simulink library "Computer_Library"  (Simulink 8.1)
settings: Solver=ode45  StartTime=0.0  StopTime=10.0  RelTol=1e-3
values from neighbouring files (symbols this model uses):
  A = 10    [CharTable.m]
  ARROW_DOWN = 48    [CharTable.m]
  ARROW_LEFT = 49    [CharTable.m]
  ARROW_RIGHT = 50    [CharTable.m]
  ARROW_UP = 47    [CharTable.m]
  ASTERISK = 39    [CharTable.m]
  B = 11    [CharTable.m]
  BACKSLASH = 43    [CharTable.m]
  C = 12    [CharTable.m]
  COLON = 40    [CharTable.m]
  COMMA = 53    [CharTable.m]
  CROSS = 38    [CharTable.m]
  CURSOR = 62    [CharTable.m]
  D = 13    [CharTable.m]
  DOT = 52    [CharTable.m]
  EQUAL = 44    [CharTable.m]
  EXCLAMATION_MARK = 55    [CharTable.m]
  F = 15    [CharTable.m]
  G = 16    [CharTable.m]
  GREATER_THAN = 46    [CharTable.m]
  H = 17    [CharTable.m]
  I = 18    [CharTable.m]
  J = 19    [CharTable.m]
  K = 20    [CharTable.m]
  L = 21    [CharTable.m]
  LEFT_PARENTHESES = 59    [CharTable.m]
  LESS_THAN = 45    [CharTable.m]
  M = 22    [CharTable.m]
  MINUS = 37    [CharTable.m]
  N = 23    [CharTable.m]
  O = 24    [CharTable.m]
  P = 25    [CharTable.m]
  PERCENT = 58    [CharTable.m]
  PLUS = 36    [CharTable.m]
  Q = 32    [CharTable.m]
  QUESTION_MARK = 54    [CharTable.m]
  QUOTE = 56    [CharTable.m]
  R = 26    [CharTable.m]
  RECTANGLE = 63    [CharTable.m]
  RIGHT_PARENTHESES = 60    [CharTable.m]
  RomCode = reshape(transpose(RomCode), [], 1)    [ROM.m]
  S = 27    [CharTable.m]
  SEMICOLON = 41    [CharTable.m]
  SHARP = 57    [CharTable.m]
  SLASH = 42    [CharTable.m]
  SPACE = 61    [CharTable.m]
  T = 28    [CharTable.m]
  U = 29    [CharTable.m]
  UNDERSCORE = 51    [CharTable.m]
  V = 30    [CharTable.m]
  W = 31    [CharTable.m]
  X = 33    [CharTable.m]
  Y = 34    [CharTable.m]
  Z = 35    [CharTable.m]
undefined symbols (not defined in the file or in its folder): char_0
libraries: Memory_Blocks_Lib x116, Byte_Multiplexers_Lib x44, commutil2 x18, Bit_Multiplexers_Lib x17, Decoders_Lib x9, simulink_extras x8, Logic_Operations_Lib x4, Byte_Demultiplexers_Lib x2, Arithmetic_Operations_Lib x2, dspsnks4 x1
(part 4 of 4)

== system Computer_Library/Character_Table/Characters(ARROW_DOWN..RECTANGLE)/Char_QUOTE ==
  Byte_01 : Constant  Value=char(2, QUOTE)  OutDataTypeStr=uint8
  Byte_02 : Constant  Value=char(3, QUOTE)  OutDataTypeStr=uint8
  Byte_03 : Constant  Value=char(4, QUOTE)  OutDataTypeStr=uint8
  Byte_04 : Constant  Value=char(5, QUOTE)  OutDataTypeStr=uint8
  Byte_05 : Constant  Value=char(6, QUOTE)  OutDataTypeStr=uint8
  Byte_06 : Constant  Value=char(7, QUOTE)  OutDataTypeStr=uint8
  Byte_07 : Constant  Value=char(8, QUOTE)  OutDataTypeStr=uint8
  Byte_1 : Constant  Value=char(1, QUOTE)  OutDataTypeStr=uint8
  Column_1(1B) : Outport
  Column_2(1B) : Outport  Port=2
  Column_3(1B) : Outport  Port=3
  Column_4(1B) : Outport  Port=4
  Column_5(1B) : Outport  Port=5
  Column_6(1B) : Outport  Port=6
  Column_7(1B) : Outport  Port=7
  Column_8(1B) : Outport  Port=8
  wires:
  Byte_05/1 -> Column_6(1B)/1
  Byte_04/1 -> Column_5(1B)/1
  Byte_01/1 -> Column_2(1B)/1
  Byte_07/1 -> Column_8(1B)/1
  Byte_03/1 -> Column_4(1B)/1
  Byte_06/1 -> Column_7(1B)/1
  Byte_1/1 -> Column_1(1B)/1
  Byte_02/1 -> Column_3(1B)/1

== system Computer_Library/Character_Table/Characters(ARROW_DOWN..RECTANGLE)/Char_RECTANGLE ==
  Byte_01 : Constant  Value=char(2, RECTANGLE)  OutDataTypeStr=uint8
  Byte_02 : Constant  Value=char(3, RECTANGLE)  OutDataTypeStr=uint8
  Byte_03 : Constant  Value=char(4, RECTANGLE)  OutDataTypeStr=uint8
  Byte_04 : Constant  Value=char(5, RECTANGLE)  OutDataTypeStr=uint8
  Byte_05 : Constant  Value=char(6, RECTANGLE)  OutDataTypeStr=uint8
  Byte_06 : Constant  Value=char(7, RECTANGLE)  OutDataTypeStr=uint8
  Byte_07 : Constant  Value=char(8, RECTANGLE)  OutDataTypeStr=uint8
  Byte_1 : Constant  Value=char(1, RECTANGLE)  OutDataTypeStr=uint8
  Column_1(1B) : Outport
  Column_2(1B) : Outport  Port=2
  Column_3(1B) : Outport  Port=3
  Column_4(1B) : Outport  Port=4
  Column_5(1B) : Outport  Port=5
  Column_6(1B) : Outport  Port=6
  Column_7(1B) : Outport  Port=7
  Column_8(1B) : Outport  Port=8
  wires:
  Byte_05/1 -> Column_6(1B)/1
  Byte_04/1 -> Column_5(1B)/1
  Byte_01/1 -> Column_2(1B)/1
  Byte_07/1 -> Column_8(1B)/1
  Byte_03/1 -> Column_4(1B)/1
  Byte_06/1 -> Column_7(1B)/1
  Byte_1/1 -> Column_1(1B)/1
  Byte_02/1 -> Column_3(1B)/1

== system Computer_Library/Character_Table/Characters(ARROW_DOWN..RECTANGLE)/Char_RIGHT_PARENTHESES ==
  Byte_01 : Constant  Value=char(2, RIGHT_PARENTHESES)  OutDataTypeStr=uint8
  Byte_02 : Constant  Value=char(3, RIGHT_PARENTHESES)  OutDataTypeStr=uint8
  Byte_03 : Constant  Value=char(4, RIGHT_PARENTHESES)  OutDataTypeStr=uint8
  Byte_04 : Constant  Value=char(5, RIGHT_PARENTHESES)  OutDataTypeStr=uint8
  Byte_05 : Constant  Value=char(6, RIGHT_PARENTHESES)  OutDataTypeStr=uint8
  Byte_06 : Constant  Value=char(7, RIGHT_PARENTHESES)  OutDataTypeStr=uint8
  Byte_07 : Constant  Value=char(8, RIGHT_PARENTHESES)  OutDataTypeStr=uint8
  Byte_1 : Constant  Value=char(1, RIGHT_PARENTHESES)  OutDataTypeStr=uint8
  Column_1(1B) : Outport
  Column_2(1B) : Outport  Port=2
  Column_3(1B) : Outport  Port=3
  Column_4(1B) : Outport  Port=4
  Column_5(1B) : Outport  Port=5
  Column_6(1B) : Outport  Port=6
  Column_7(1B) : Outport  Port=7
  Column_8(1B) : Outport  Port=8
  wires:
  Byte_05/1 -> Column_6(1B)/1
  Byte_04/1 -> Column_5(1B)/1
  Byte_01/1 -> Column_2(1B)/1
  Byte_07/1 -> Column_8(1B)/1
  Byte_03/1 -> Column_4(1B)/1
  Byte_06/1 -> Column_7(1B)/1
  Byte_1/1 -> Column_1(1B)/1
  Byte_02/1 -> Column_3(1B)/1

== system Computer_Library/Character_Table/Characters(ARROW_DOWN..RECTANGLE)/Char_SHARP ==
  Byte_01 : Constant  Value=char(2, SHARP)  OutDataTypeStr=uint8
  Byte_02 : Constant  Value=char(3, SHARP)  OutDataTypeStr=uint8
  Byte_03 : Constant  Value=char(4, SHARP)  OutDataTypeStr=uint8
  Byte_04 : Constant  Value=char(5, SHARP)  OutDataTypeStr=uint8
  Byte_05 : Constant  Value=char(6, SHARP)  OutDataTypeStr=uint8
  Byte_06 : Constant  Value=char(7, SHARP)  OutDataTypeStr=uint8
  Byte_07 : Constant  Value=char(8, SHARP)  OutDataTypeStr=uint8
  Byte_1 : Constant  Value=char(1, SHARP)  OutDataTypeStr=uint8
  Column_1(1B) : Outport
  Column_2(1B) : Outport  Port=2
  Column_3(1B) : Outport  Port=3
  Column_4(1B) : Outport  Port=4
  Column_5(1B) : Outport  Port=5
  Column_6(1B) : Outport  Port=6
  Column_7(1B) : Outport  Port=7
  Column_8(1B) : Outport  Port=8
  wires:
  Byte_05/1 -> Column_6(1B)/1
  Byte_04/1 -> Column_5(1B)/1
  Byte_01/1 -> Column_2(1B)/1
  Byte_07/1 -> Column_8(1B)/1
  Byte_03/1 -> Column_4(1B)/1
  Byte_06/1 -> Column_7(1B)/1
  Byte_1/1 -> Column_1(1B)/1
  Byte_02/1 -> Column_3(1B)/1

== system Computer_Library/Character_Table/Characters(ARROW_DOWN..RECTANGLE)/Char_SPACE ==
  Byte_01 : Constant  Value=char(2, SPACE)  OutDataTypeStr=uint8
  Byte_02 : Constant  Value=char(3, SPACE)  OutDataTypeStr=uint8
  Byte_03 : Constant  Value=char(4, SPACE)  OutDataTypeStr=uint8
  Byte_04 : Constant  Value=char(5, SPACE)  OutDataTypeStr=uint8
  Byte_05 : Constant  Value=char(6, SPACE)  OutDataTypeStr=uint8
  Byte_06 : Constant  Value=char(7, SPACE)  OutDataTypeStr=uint8
  Byte_07 : Constant  Value=char(8, SPACE)  OutDataTypeStr=uint8
  Byte_1 : Constant  Value=char(1, SPACE)  OutDataTypeStr=uint8
  Column_1(1B) : Outport
  Column_2(1B) : Outport  Port=2
  Column_3(1B) : Outport  Port=3
  Column_4(1B) : Outport  Port=4
  Column_5(1B) : Outport  Port=5
  Column_6(1B) : Outport  Port=6
  Column_7(1B) : Outport  Port=7
  Column_8(1B) : Outport  Port=8
  wires:
  Byte_05/1 -> Column_6(1B)/1
  Byte_04/1 -> Column_5(1B)/1
  Byte_01/1 -> Column_2(1B)/1
  Byte_07/1 -> Column_8(1B)/1
  Byte_03/1 -> Column_4(1B)/1
  Byte_06/1 -> Column_7(1B)/1
  Byte_1/1 -> Column_1(1B)/1
  Byte_02/1 -> Column_3(1B)/1

== system Computer_Library/Character_Table/Characters(ARROW_DOWN..RECTANGLE)/Char_UNDERSCORE ==
  Byte_01 : Constant  Value=char(2, UNDERSCORE)  OutDataTypeStr=uint8
  Byte_02 : Constant  Value=char(3, UNDERSCORE)  OutDataTypeStr=uint8
  Byte_03 : Constant  Value=char(4, UNDERSCORE)  OutDataTypeStr=uint8
  Byte_04 : Constant  Value=char(5, UNDERSCORE)  OutDataTypeStr=uint8
  Byte_05 : Constant  Value=char(6, UNDERSCORE)  OutDataTypeStr=uint8
  Byte_06 : Constant  Value=char(7, UNDERSCORE)  OutDataTypeStr=uint8
  Byte_07 : Constant  Value=char(8, UNDERSCORE)  OutDataTypeStr=uint8
  Byte_1 : Constant  Value=char(1, UNDERSCORE)  OutDataTypeStr=uint8
  Column_1(1B) : Outport
  Column_2(1B) : Outport  Port=2
  Column_3(1B) : Outport  Port=3
  Column_4(1B) : Outport  Port=4
  Column_5(1B) : Outport  Port=5
  Column_6(1B) : Outport  Port=6
  Column_7(1B) : Outport  Port=7
  Column_8(1B) : Outport  Port=8
  wires:
  Byte_05/1 -> Column_6(1B)/1
  Byte_04/1 -> Column_5(1B)/1
  Byte_01/1 -> Column_2(1B)/1
  Byte_07/1 -> Column_8(1B)/1
  Byte_03/1 -> Column_4(1B)/1
  Byte_06/1 -> Column_7(1B)/1
  Byte_1/1 -> Column_1(1B)/1
  Byte_02/1 -> Column_3(1B)/1

== system Computer_Library/Character_Table/Characters(G..W)/Char_G ==
  Byte_01 : Constant  Value=char(2, G)  OutDataTypeStr=uint8
  Byte_02 : Constant  Value=char(3, G)  OutDataTypeStr=uint8
  Byte_03 : Constant  Value=char(4, G)  OutDataTypeStr=uint8
  Byte_04 : Constant  Value=char(5, G)  OutDataTypeStr=uint8
  Byte_05 : Constant  Value=char(6, G)  OutDataTypeStr=uint8
  Byte_06 : Constant  Value=char(7, G)  OutDataTypeStr=uint8
  Byte_07 : Constant  Value=char(8, G)  OutDataTypeStr=uint8
  Byte_1 : Constant  Value=char(1, G)  OutDataTypeStr=uint8
  Column_1(1B) : Outport
  Column_2(1B) : Outport  Port=2
  Column_3(1B) : Outport  Port=3
  Column_4(1B) : Outport  Port=4
  Column_5(1B) : Outport  Port=5
  Column_6(1B) : Outport  Port=6
  Column_7(1B) : Outport  Port=7
  Column_8(1B) : Outport  Port=8
  wires:
  Byte_05/1 -> Column_6(1B)/1
  Byte_04/1 -> Column_5(1B)/1
  Byte_01/1 -> Column_2(1B)/1
  Byte_07/1 -> Column_8(1B)/1
  Byte_03/1 -> Column_4(1B)/1
  Byte_06/1 -> Column_7(1B)/1
  Byte_1/1 -> Column_1(1B)/1
  Byte_02/1 -> Column_3(1B)/1

== system Computer_Library/Character_Table/Characters(G..W)/Char_H ==
  Byte_01 : Constant  Value=char(2, H)  OutDataTypeStr=uint8
  Byte_02 : Constant  Value=char(3, H)  OutDataTypeStr=uint8
  Byte_03 : Constant  Value=char(4, H)  OutDataTypeStr=uint8
  Byte_04 : Constant  Value=char(5, H)  OutDataTypeStr=uint8
  Byte_05 : Constant  Value=char(6, H)  OutDataTypeStr=uint8
  Byte_06 : Constant  Value=char(7, H)  OutDataTypeStr=uint8
  Byte_07 : Constant  Value=char(8, H)  OutDataTypeStr=uint8
  Byte_1 : Constant  Value=char(1, H)  OutDataTypeStr=uint8
  Column_1(1B) : Outport
  Column_2(1B) : Outport  Port=2
  Column_3(1B) : Outport  Port=3
  Column_4(1B) : Outport  Port=4
  Column_5(1B) : Outport  Port=5
  Column_6(1B) : Outport  Port=6
  Column_7(1B) : Outport  Port=7
  Column_8(1B) : Outport  Port=8
  wires:
  Byte_05/1 -> Column_6(1B)/1
  Byte_04/1 -> Column_5(1B)/1
  Byte_01/1 -> Column_2(1B)/1
  Byte_07/1 -> Column_8(1B)/1
  Byte_03/1 -> Column_4(1B)/1
  Byte_06/1 -> Column_7(1B)/1
  Byte_1/1 -> Column_1(1B)/1
  Byte_02/1 -> Column_3(1B)/1

== system Computer_Library/Character_Table/Characters(G..W)/Char_I ==
  Byte_01 : Constant  Value=char(2, I)  OutDataTypeStr=uint8
  Byte_02 : Constant  Value=char(3, I)  OutDataTypeStr=uint8
  Byte_03 : Constant  Value=char(4, I)  OutDataTypeStr=uint8
  Byte_04 : Constant  Value=char(5, I)  OutDataTypeStr=uint8
  Byte_05 : Constant  Value=char(6, I)  OutDataTypeStr=uint8
  Byte_06 : Constant  Value=char(7, I)  OutDataTypeStr=uint8
  Byte_07 : Constant  Value=char(8, I)  OutDataTypeStr=uint8
  Byte_1 : Constant  Value=char(1, I)  OutDataTypeStr=uint8
  Column_1(1B) : Outport
  Column_2(1B) : Outport  Port=2
  Column_3(1B) : Outport  Port=3
  Column_4(1B) : Outport  Port=4
  Column_5(1B) : Outport  Port=5
  Column_6(1B) : Outport  Port=6
  Column_7(1B) : Outport  Port=7
  Column_8(1B) : Outport  Port=8
  wires:
  Byte_05/1 -> Column_6(1B)/1
  Byte_04/1 -> Column_5(1B)/1
  Byte_01/1 -> Column_2(1B)/1
  Byte_07/1 -> Column_8(1B)/1
  Byte_03/1 -> Column_4(1B)/1
  Byte_06/1 -> Column_7(1B)/1
  Byte_1/1 -> Column_1(1B)/1
  Byte_02/1 -> Column_3(1B)/1

== system Computer_Library/Character_Table/Characters(G..W)/Char_J ==
  Byte_01 : Constant  Value=char(2, J)  OutDataTypeStr=uint8
  Byte_02 : Constant  Value=char(3, J)  OutDataTypeStr=uint8
  Byte_03 : Constant  Value=char(4, J)  OutDataTypeStr=uint8
  Byte_04 : Constant  Value=char(5, J)  OutDataTypeStr=uint8
  Byte_05 : Constant  Value=char(6, J)  OutDataTypeStr=uint8
  Byte_06 : Constant  Value=char(7, J)  OutDataTypeStr=uint8
  Byte_07 : Constant  Value=char(8, J)  OutDataTypeStr=uint8
  Byte_1 : Constant  Value=char(1, J)  OutDataTypeStr=uint8
  Column_1(1B) : Outport
  Column_2(1B) : Outport  Port=2
  Column_3(1B) : Outport  Port=3
  Column_4(1B) : Outport  Port=4
  Column_5(1B) : Outport  Port=5
  Column_6(1B) : Outport  Port=6
  Column_7(1B) : Outport  Port=7
  Column_8(1B) : Outport  Port=8
  wires:
  Byte_05/1 -> Column_6(1B)/1
  Byte_04/1 -> Column_5(1B)/1
  Byte_01/1 -> Column_2(1B)/1
  Byte_07/1 -> Column_8(1B)/1
  Byte_03/1 -> Column_4(1B)/1
  Byte_06/1 -> Column_7(1B)/1
  Byte_1/1 -> Column_1(1B)/1
  Byte_02/1 -> Column_3(1B)/1

== system Computer_Library/Character_Table/Characters(G..W)/Char_K ==
  Byte_01 : Constant  Value=char(2, K)  OutDataTypeStr=uint8
  Byte_02 : Constant  Value=char(3, K)  OutDataTypeStr=uint8
  Byte_03 : Constant  Value=char(4, K)  OutDataTypeStr=uint8
  Byte_04 : Constant  Value=char(5, K)  OutDataTypeStr=uint8
  Byte_05 : Constant  Value=char(6, K)  OutDataTypeStr=uint8
  Byte_06 : Constant  Value=char(7, K)  OutDataTypeStr=uint8
  Byte_07 : Constant  Value=char(8, K)  OutDataTypeStr=uint8
  Byte_1 : Constant  Value=char(1, K)  OutDataTypeStr=uint8
  Column_1(1B) : Outport
  Column_2(1B) : Outport  Port=2
  Column_3(1B) : Outport  Port=3
  Column_4(1B) : Outport  Port=4
  Column_5(1B) : Outport  Port=5
  Column_6(1B) : Outport  Port=6
  Column_7(1B) : Outport  Port=7
  Column_8(1B) : Outport  Port=8
  wires:
  Byte_05/1 -> Column_6(1B)/1
  Byte_04/1 -> Column_5(1B)/1
  Byte_01/1 -> Column_2(1B)/1
  Byte_07/1 -> Column_8(1B)/1
  Byte_03/1 -> Column_4(1B)/1
  Byte_06/1 -> Column_7(1B)/1
  Byte_1/1 -> Column_1(1B)/1
  Byte_02/1 -> Column_3(1B)/1

== system Computer_Library/Character_Table/Characters(G..W)/Char_L ==
  Byte_01 : Constant  Value=char(2, L)  OutDataTypeStr=uint8
  Byte_02 : Constant  Value=char(3, L)  OutDataTypeStr=uint8
  Byte_03 : Constant  Value=char(4, L)  OutDataTypeStr=uint8
  Byte_04 : Constant  Value=char(5, L)  OutDataTypeStr=uint8
  Byte_05 : Constant  Value=char(6, L)  OutDataTypeStr=uint8
  Byte_06 : Constant  Value=char(7, L)  OutDataTypeStr=uint8
  Byte_07 : Constant  Value=char(8, L)  OutDataTypeStr=uint8
  Byte_1 : Constant  Value=char(1, L)  OutDataTypeStr=uint8
  Column_1(1B) : Outport
  Column_2(1B) : Outport  Port=2
  Column_3(1B) : Outport  Port=3
  Column_4(1B) : Outport  Port=4
  Column_5(1B) : Outport  Port=5
  Column_6(1B) : Outport  Port=6
  Column_7(1B) : Outport  Port=7
  Column_8(1B) : Outport  Port=8
  wires:
  Byte_05/1 -> Column_6(1B)/1
  Byte_04/1 -> Column_5(1B)/1
  Byte_01/1 -> Column_2(1B)/1
  Byte_07/1 -> Column_8(1B)/1
  Byte_03/1 -> Column_4(1B)/1
  Byte_06/1 -> Column_7(1B)/1
  Byte_1/1 -> Column_1(1B)/1
  Byte_02/1 -> Column_3(1B)/1

== system Computer_Library/Character_Table/Characters(G..W)/Char_M ==
  Byte_01 : Constant  Value=char(2, M)  OutDataTypeStr=uint8
  Byte_02 : Constant  Value=char(3, M)  OutDataTypeStr=uint8
  Byte_03 : Constant  Value=char(4, M)  OutDataTypeStr=uint8
  Byte_04 : Constant  Value=char(5, M)  OutDataTypeStr=uint8
  Byte_05 : Constant  Value=char(6, M)  OutDataTypeStr=uint8
  Byte_06 : Constant  Value=char(7, M)  OutDataTypeStr=uint8
  Byte_07 : Constant  Value=char(8, M)  OutDataTypeStr=uint8
  Byte_1 : Constant  Value=char(1, M)  OutDataTypeStr=uint8
  Column_1(1B) : Outport
  Column_2(1B) : Outport  Port=2
  Column_3(1B) : Outport  Port=3
  Column_4(1B) : Outport  Port=4
  Column_5(1B) : Outport  Port=5
  Column_6(1B) : Outport  Port=6
  Column_7(1B) : Outport  Port=7
  Column_8(1B) : Outport  Port=8
  wires:
  Byte_05/1 -> Column_6(1B)/1
  Byte_04/1 -> Column_5(1B)/1
  Byte_01/1 -> Column_2(1B)/1
  Byte_07/1 -> Column_8(1B)/1
  Byte_03/1 -> Column_4(1B)/1
  Byte_06/1 -> Column_7(1B)/1
  Byte_1/1 -> Column_1(1B)/1
  Byte_02/1 -> Column_3(1B)/1

== system Computer_Library/Character_Table/Characters(G..W)/Char_N ==
  Byte_01 : Constant  Value=char(2, N)  OutDataTypeStr=uint8
  Byte_02 : Constant  Value=char(3, N)  OutDataTypeStr=uint8
  Byte_03 : Constant  Value=char(4, N)  OutDataTypeStr=uint8
  Byte_04 : Constant  Value=char(5, N)  OutDataTypeStr=uint8
  Byte_05 : Constant  Value=char(6, N)  OutDataTypeStr=uint8
  Byte_06 : Constant  Value=char(7, N)  OutDataTypeStr=uint8
  Byte_07 : Constant  Value=char(8, N)  OutDataTypeStr=uint8
  Byte_1 : Constant  Value=char(1, N)  OutDataTypeStr=uint8
  Column_1(1B) : Outport
  Column_2(1B) : Outport  Port=2
  Column_3(1B) : Outport  Port=3
  Column_4(1B) : Outport  Port=4
  Column_5(1B) : Outport  Port=5
  Column_6(1B) : Outport  Port=6
  Column_7(1B) : Outport  Port=7
  Column_8(1B) : Outport  Port=8
  wires:
  Byte_05/1 -> Column_6(1B)/1
  Byte_04/1 -> Column_5(1B)/1
  Byte_01/1 -> Column_2(1B)/1
  Byte_07/1 -> Column_8(1B)/1
  Byte_03/1 -> Column_4(1B)/1
  Byte_06/1 -> Column_7(1B)/1
  Byte_1/1 -> Column_1(1B)/1
  Byte_02/1 -> Column_3(1B)/1

== system Computer_Library/Character_Table/Characters(G..W)/Char_O ==
  Byte_01 : Constant  Value=char(2, O)  OutDataTypeStr=uint8
  Byte_02 : Constant  Value=char(3, O)  OutDataTypeStr=uint8
  Byte_03 : Constant  Value=char(4, O)  OutDataTypeStr=uint8
  Byte_04 : Constant  Value=char(5, O)  OutDataTypeStr=uint8
  Byte_05 : Constant  Value=char(6, O)  OutDataTypeStr=uint8
  Byte_06 : Constant  Value=char(7, O)  OutDataTypeStr=uint8
  Byte_07 : Constant  Value=char(8, O)  OutDataTypeStr=uint8
  Byte_1 : Constant  Value=char(1, O)  OutDataTypeStr=uint8
  Column_1(1B) : Outport
  Column_2(1B) : Outport  Port=2
  Column_3(1B) : Outport  Port=3
  Column_4(1B) : Outport  Port=4
  Column_5(1B) : Outport  Port=5
  Column_6(1B) : Outport  Port=6
  Column_7(1B) : Outport  Port=7
  Column_8(1B) : Outport  Port=8
  wires:
  Byte_05/1 -> Column_6(1B)/1
  Byte_04/1 -> Column_5(1B)/1
  Byte_01/1 -> Column_2(1B)/1
  Byte_07/1 -> Column_8(1B)/1
  Byte_03/1 -> Column_4(1B)/1
  Byte_06/1 -> Column_7(1B)/1
  Byte_1/1 -> Column_1(1B)/1
  Byte_02/1 -> Column_3(1B)/1

== system Computer_Library/Character_Table/Characters(G..W)/Char_P ==
  Byte_01 : Constant  Value=char(2, P)  OutDataTypeStr=uint8
  Byte_02 : Constant  Value=char(3, P)  OutDataTypeStr=uint8
  Byte_03 : Constant  Value=char(4, P)  OutDataTypeStr=uint8
  Byte_04 : Constant  Value=char(5, P)  OutDataTypeStr=uint8
  Byte_05 : Constant  Value=char(6, P)  OutDataTypeStr=uint8
  Byte_06 : Constant  Value=char(7, P)  OutDataTypeStr=uint8
  Byte_07 : Constant  Value=char(8, P)  OutDataTypeStr=uint8
  Byte_1 : Constant  Value=char(1, P)  OutDataTypeStr=uint8
  Column_1(1B) : Outport
  Column_2(1B) : Outport  Port=2
  Column_3(1B) : Outport  Port=3
  Column_4(1B) : Outport  Port=4
  Column_5(1B) : Outport  Port=5
  Column_6(1B) : Outport  Port=6
  Column_7(1B) : Outport  Port=7
  Column_8(1B) : Outport  Port=8
  wires:
  Byte_05/1 -> Column_6(1B)/1
  Byte_04/1 -> Column_5(1B)/1
  Byte_01/1 -> Column_2(1B)/1
  Byte_07/1 -> Column_8(1B)/1
  Byte_03/1 -> Column_4(1B)/1
  Byte_06/1 -> Column_7(1B)/1
  Byte_1/1 -> Column_1(1B)/1
  Byte_02/1 -> Column_3(1B)/1

== system Computer_Library/Character_Table/Characters(G..W)/Char_R ==
  Byte_01 : Constant  Value=char(2, R)  OutDataTypeStr=uint8
  Byte_02 : Constant  Value=char(3, R)  OutDataTypeStr=uint8
  Byte_03 : Constant  Value=char(4, R)  OutDataTypeStr=uint8
  Byte_04 : Constant  Value=char(5, R)  OutDataTypeStr=uint8
  Byte_05 : Constant  Value=char(6, R)  OutDataTypeStr=uint8
  Byte_06 : Constant  Value=char(7, R)  OutDataTypeStr=uint8
  Byte_07 : Constant  Value=char(8, R)  OutDataTypeStr=uint8
  Byte_1 : Constant  Value=char(1, R)  OutDataTypeStr=uint8
  Column_1(1B) : Outport
  Column_2(1B) : Outport  Port=2
  Column_3(1B) : Outport  Port=3
  Column_4(1B) : Outport  Port=4
  Column_5(1B) : Outport  Port=5
  Column_6(1B) : Outport  Port=6
  Column_7(1B) : Outport  Port=7
  Column_8(1B) : Outport  Port=8
  wires:
  Byte_05/1 -> Column_6(1B)/1
  Byte_04/1 -> Column_5(1B)/1
  Byte_01/1 -> Column_2(1B)/1
  Byte_07/1 -> Column_8(1B)/1
  Byte_03/1 -> Column_4(1B)/1
  Byte_06/1 -> Column_7(1B)/1
  Byte_1/1 -> Column_1(1B)/1
  Byte_02/1 -> Column_3(1B)/1

== system Computer_Library/Character_Table/Characters(G..W)/Char_S ==
  Byte_01 : Constant  Value=char(2, S)  OutDataTypeStr=uint8
  Byte_02 : Constant  Value=char(3, S)  OutDataTypeStr=uint8
  Byte_03 : Constant  Value=char(4, S)  OutDataTypeStr=uint8
  Byte_04 : Constant  Value=char(5, S)  OutDataTypeStr=uint8
  Byte_05 : Constant  Value=char(6, S)  OutDataTypeStr=uint8
  Byte_06 : Constant  Value=char(7, S)  OutDataTypeStr=uint8
  Byte_07 : Constant  Value=char(8, S)  OutDataTypeStr=uint8
  Byte_1 : Constant  Value=char(1, S)  OutDataTypeStr=uint8
  Column_1(1B) : Outport
  Column_2(1B) : Outport  Port=2
  Column_3(1B) : Outport  Port=3
  Column_4(1B) : Outport  Port=4
  Column_5(1B) : Outport  Port=5
  Column_6(1B) : Outport  Port=6
  Column_7(1B) : Outport  Port=7
  Column_8(1B) : Outport  Port=8
  wires:
  Byte_05/1 -> Column_6(1B)/1
  Byte_04/1 -> Column_5(1B)/1
  Byte_01/1 -> Column_2(1B)/1
  Byte_07/1 -> Column_8(1B)/1
  Byte_03/1 -> Column_4(1B)/1
  Byte_06/1 -> Column_7(1B)/1
  Byte_1/1 -> Column_1(1B)/1
  Byte_02/1 -> Column_3(1B)/1

== system Computer_Library/Character_Table/Characters(G..W)/Char_T ==
  Byte_01 : Constant  Value=char(2, T)  OutDataTypeStr=uint8
  Byte_02 : Constant  Value=char(3, T)  OutDataTypeStr=uint8
  Byte_03 : Constant  Value=char(4, T)  OutDataTypeStr=uint8
  Byte_04 : Constant  Value=char(5, T)  OutDataTypeStr=uint8
  Byte_05 : Constant  Value=char(6, T)  OutDataTypeStr=uint8
  Byte_06 : Constant  Value=char(7, T)  OutDataTypeStr=uint8
  Byte_07 : Constant  Value=char(8, T)  OutDataTypeStr=uint8
  Byte_1 : Constant  Value=char(1, T)  OutDataTypeStr=uint8
  Column_1(1B) : Outport
  Column_2(1B) : Outport  Port=2
  Column_3(1B) : Outport  Port=3
  Column_4(1B) : Outport  Port=4
  Column_5(1B) : Outport  Port=5
  Column_6(1B) : Outport  Port=6
  Column_7(1B) : Outport  Port=7
  Column_8(1B) : Outport  Port=8
  wires:
  Byte_05/1 -> Column_6(1B)/1
  Byte_04/1 -> Column_5(1B)/1
  Byte_01/1 -> Column_2(1B)/1
  Byte_07/1 -> Column_8(1B)/1
  Byte_03/1 -> Column_4(1B)/1
  Byte_06/1 -> Column_7(1B)/1
  Byte_1/1 -> Column_1(1B)/1
  Byte_02/1 -> Column_3(1B)/1

== system Computer_Library/Character_Table/Characters(G..W)/Char_U ==
  Byte_01 : Constant  Value=char(2, U)  OutDataTypeStr=uint8
  Byte_02 : Constant  Value=char(3, U)  OutDataTypeStr=uint8
  Byte_03 : Constant  Value=char(4, U)  OutDataTypeStr=uint8
  Byte_04 : Constant  Value=char(5, U)  OutDataTypeStr=uint8
  Byte_05 : Constant  Value=char(6, U)  OutDataTypeStr=uint8
  Byte_06 : Constant  Value=char(7, U)  OutDataTypeStr=uint8
  Byte_07 : Constant  Value=char(8, U)  OutDataTypeStr=uint8
  Byte_1 : Constant  Value=char(1, U)  OutDataTypeStr=uint8
  Column_1(1B) : Outport
  Column_2(1B) : Outport  Port=2
  Column_3(1B) : Outport  Port=3
  Column_4(1B) : Outport  Port=4
  Column_5(1B) : Outport  Port=5
  Column_6(1B) : Outport  Port=6
  Column_7(1B) : Outport  Port=7
  Column_8(1B) : Outport  Port=8
  wires:
  Byte_05/1 -> Column_6(1B)/1
  Byte_04/1 -> Column_5(1B)/1
  Byte_01/1 -> Column_2(1B)/1
  Byte_07/1 -> Column_8(1B)/1
  Byte_03/1 -> Column_4(1B)/1
  Byte_06/1 -> Column_7(1B)/1
  Byte_1/1 -> Column_1(1B)/1
  Byte_02/1 -> Column_3(1B)/1

== system Computer_Library/Character_Table/Characters(G..W)/Char_V ==
  Byte_01 : Constant  Value=char(2, V)  OutDataTypeStr=uint8
  Byte_02 : Constant  Value=char(3, V)  OutDataTypeStr=uint8
  Byte_03 : Constant  Value=char(4, V)  OutDataTypeStr=uint8
  Byte_04 : Constant  Value=char(5, V)  OutDataTypeStr=uint8
  Byte_05 : Constant  Value=char(6, V)  OutDataTypeStr=uint8
  Byte_06 : Constant  Value=char(7, V)  OutDataTypeStr=uint8
  Byte_07 : Constant  Value=char(8, V)  OutDataTypeStr=uint8
  Byte_1 : Constant  Value=char(1, V)  OutDataTypeStr=uint8
  Column_1(1B) : Outport
  Column_2(1B) : Outport  Port=2
  Column_3(1B) : Outport  Port=3
  Column_4(1B) : Outport  Port=4
  Column_5(1B) : Outport  Port=5
  Column_6(1B) : Outport  Port=6
  Column_7(1B) : Outport  Port=7
  Column_8(1B) : Outport  Port=8
  wires:
  Byte_05/1 -> Column_6(1B)/1
  Byte_04/1 -> Column_5(1B)/1
  Byte_01/1 -> Column_2(1B)/1
  Byte_07/1 -> Column_8(1B)/1
  Byte_03/1 -> Column_4(1B)/1
  Byte_06/1 -> Column_7(1B)/1
  Byte_1/1 -> Column_1(1B)/1
  Byte_02/1 -> Column_3(1B)/1

== system Computer_Library/Character_Table/Characters(G..W)/Char_W ==
  Byte_01 : Constant  Value=char(2, W)  OutDataTypeStr=uint8
  Byte_02 : Constant  Value=char(3, W)  OutDataTypeStr=uint8
  Byte_03 : Constant  Value=char(4, W)  OutDataTypeStr=uint8
  Byte_04 : Constant  Value=char(5, W)  OutDataTypeStr=uint8
  Byte_05 : Constant  Value=char(6, W)  OutDataTypeStr=uint8
  Byte_06 : Constant  Value=char(7, W)  OutDataTypeStr=uint8
  Byte_07 : Constant  Value=char(8, W)  OutDataTypeStr=uint8
  Byte_1 : Constant  Value=char(1, W)  OutDataTypeStr=uint8
  Column_1(1B) : Outport
  Column_2(1B) : Outport  Port=2
  Column_3(1B) : Outport  Port=3
  Column_4(1B) : Outport  Port=4
  Column_5(1B) : Outport  Port=5
  Column_6(1B) : Outport  Port=6
  Column_7(1B) : Outport  Port=7
  Column_8(1B) : Outport  Port=8
  wires:
  Byte_05/1 -> Column_6(1B)/1
  Byte_04/1 -> Column_5(1B)/1
  Byte_01/1 -> Column_2(1B)/1
  Byte_07/1 -> Column_8(1B)/1
  Byte_03/1 -> Column_4(1B)/1
  Byte_06/1 -> Column_7(1B)/1
  Byte_1/1 -> Column_1(1B)/1
  Byte_02/1 -> Column_3(1B)/1

== system Computer_Library/Character_Table/Characters(Q..ARROW_UP)/Char_ARROW_UP ==
  Byte_01 : Constant  Value=char(2, ARROW_UP)  OutDataTypeStr=uint8
  Byte_02 : Constant  Value=char(3, ARROW_UP)  OutDataTypeStr=uint8
  Byte_03 : Constant  Value=char(4, ARROW_UP)  OutDataTypeStr=uint8
  Byte_04 : Constant  Value=char(5, ARROW_UP)  OutDataTypeStr=uint8
  Byte_05 : Constant  Value=char(6, ARROW_UP)  OutDataTypeStr=uint8
  Byte_06 : Constant  Value=char(7, ARROW_UP)  OutDataTypeStr=uint8
  Byte_07 : Constant  Value=char(8, ARROW_UP)  OutDataTypeStr=uint8
  Byte_1 : Constant  Value=char(1, ARROW_UP)  OutDataTypeStr=uint8
  Column_1(1B) : Outport
  Column_2(1B) : Outport  Port=2
  Column_3(1B) : Outport  Port=3
  Column_4(1B) : Outport  Port=4
  Column_5(1B) : Outport  Port=5
  Column_6(1B) : Outport  Port=6
  Column_7(1B) : Outport  Port=7
  Column_8(1B) : Outport  Port=8
  wires:
  Byte_05/1 -> Column_6(1B)/1
  Byte_04/1 -> Column_5(1B)/1
  Byte_01/1 -> Column_2(1B)/1
  Byte_07/1 -> Column_8(1B)/1
  Byte_03/1 -> Column_4(1B)/1
  Byte_06/1 -> Column_7(1B)/1
  Byte_1/1 -> Column_1(1B)/1
  Byte_02/1 -> Column_3(1B)/1

== system Computer_Library/Character_Table/Characters(Q..ARROW_UP)/Char_ASTERISK ==
  Byte_01 : Constant  Value=char(2, ASTERISK)  OutDataTypeStr=uint8
  Byte_02 : Constant  Value=char(3, ASTERISK)  OutDataTypeStr=uint8
  Byte_03 : Constant  Value=char(4, ASTERISK)  OutDataTypeStr=uint8
  Byte_04 : Constant  Value=char(5, ASTERISK)  OutDataTypeStr=uint8
  Byte_05 : Constant  Value=char(6, ASTERISK)  OutDataTypeStr=uint8
  Byte_06 : Constant  Value=char(7, ASTERISK)  OutDataTypeStr=uint8
  Byte_07 : Constant  Value=char(8, ASTERISK)  OutDataTypeStr=uint8
  Byte_1 : Constant  Value=char(1, ASTERISK)  OutDataTypeStr=uint8
  Column_1(1B) : Outport
  Column_2(1B) : Outport  Port=2
  Column_3(1B) : Outport  Port=3
  Column_4(1B) : Outport  Port=4
  Column_5(1B) : Outport  Port=5
  Column_6(1B) : Outport  Port=6
  Column_7(1B) : Outport  Port=7
  Column_8(1B) : Outport  Port=8
  wires:
  Byte_05/1 -> Column_6(1B)/1
  Byte_04/1 -> Column_5(1B)/1
  Byte_01/1 -> Column_2(1B)/1
  Byte_07/1 -> Column_8(1B)/1
  Byte_03/1 -> Column_4(1B)/1
  Byte_06/1 -> Column_7(1B)/1
  Byte_1/1 -> Column_1(1B)/1
  Byte_02/1 -> Column_3(1B)/1

== system Computer_Library/Character_Table/Characters(Q..ARROW_UP)/Char_BACKSLASH ==
  Byte_01 : Constant  Value=char(2, BACKSLASH)  OutDataTypeStr=uint8
  Byte_02 : Constant  Value=char(3, BACKSLASH)  OutDataTypeStr=uint8
  Byte_03 : Constant  Value=char(4, BACKSLASH)  OutDataTypeStr=uint8
  Byte_04 : Constant  Value=char(5, BACKSLASH)  OutDataTypeStr=uint8
  Byte_05 : Constant  Value=char(6, BACKSLASH)  OutDataTypeStr=uint8
  Byte_06 : Constant  Value=char(7, BACKSLASH)  OutDataTypeStr=uint8
  Byte_07 : Constant  Value=char(8, BACKSLASH)  OutDataTypeStr=uint8
  Byte_1 : Constant  Value=char(1, BACKSLASH)  OutDataTypeStr=uint8
  Column_1(1B) : Outport
  Column_2(1B) : Outport  Port=2
  Column_3(1B) : Outport  Port=3
  Column_4(1B) : Outport  Port=4
  Column_5(1B) : Outport  Port=5
  Column_6(1B) : Outport  Port=6
  Column_7(1B) : Outport  Port=7
  Column_8(1B) : Outport  Port=8
  wires:
  Byte_05/1 -> Column_6(1B)/1
  Byte_04/1 -> Column_5(1B)/1
  Byte_01/1 -> Column_2(1B)/1
  Byte_07/1 -> Column_8(1B)/1
  Byte_03/1 -> Column_4(1B)/1
  Byte_06/1 -> Column_7(1B)/1
  Byte_1/1 -> Column_1(1B)/1
  Byte_02/1 -> Column_3(1B)/1

== system Computer_Library/Character_Table/Characters(Q..ARROW_UP)/Char_COLON ==
  Byte_01 : Constant  Value=char(2, COLON)  OutDataTypeStr=uint8
  Byte_02 : Constant  Value=char(3, COLON)  OutDataTypeStr=uint8
  Byte_03 : Constant  Value=char(4, COLON)  OutDataTypeStr=uint8
  Byte_04 : Constant  Value=char(5, COLON)  OutDataTypeStr=uint8
  Byte_05 : Constant  Value=char(6, COLON)  OutDataTypeStr=uint8
  Byte_06 : Constant  Value=char(7, COLON)  OutDataTypeStr=uint8
  Byte_07 : Constant  Value=char(8, COLON)  OutDataTypeStr=uint8
  Byte_1 : Constant  Value=char(1, COLON)  OutDataTypeStr=uint8
  Column_1(1B) : Outport
  Column_2(1B) : Outport  Port=2
  Column_3(1B) : Outport  Port=3
  Column_4(1B) : Outport  Port=4
  Column_5(1B) : Outport  Port=5
  Column_6(1B) : Outport  Port=6
  Column_7(1B) : Outport  Port=7
  Column_8(1B) : Outport  Port=8
  wires:
  Byte_05/1 -> Column_6(1B)/1
  Byte_04/1 -> Column_5(1B)/1
  Byte_01/1 -> Column_2(1B)/1
  Byte_07/1 -> Column_8(1B)/1
  Byte_03/1 -> Column_4(1B)/1
  Byte_06/1 -> Column_7(1B)/1
  Byte_1/1 -> Column_1(1B)/1
  Byte_02/1 -> Column_3(1B)/1

== system Computer_Library/Character_Table/Characters(Q..ARROW_UP)/Char_CROSS ==
  Byte_01 : Constant  Value=char(2, CROSS)  OutDataTypeStr=uint8
  Byte_02 : Constant  Value=char(3, CROSS)  OutDataTypeStr=uint8
  Byte_03 : Constant  Value=char(4, CROSS)  OutDataTypeStr=uint8
  Byte_04 : Constant  Value=char(5, CROSS)  OutDataTypeStr=uint8
  Byte_05 : Constant  Value=char(6, CROSS)  OutDataTypeStr=uint8
  Byte_06 : Constant  Value=char(7, CROSS)  OutDataTypeStr=uint8
  Byte_07 : Constant  Value=char(8, CROSS)  OutDataTypeStr=uint8
  Byte_1 : Constant  Value=char(1, CROSS)  OutDataTypeStr=uint8
  Column_1(1B) : Outport
  Column_2(1B) : Outport  Port=2
  Column_3(1B) : Outport  Port=3
  Column_4(1B) : Outport  Port=4
  Column_5(1B) : Outport  Port=5
  Column_6(1B) : Outport  Port=6
  Column_7(1B) : Outport  Port=7
  Column_8(1B) : Outport  Port=8
  wires:
  Byte_05/1 -> Column_6(1B)/1
  Byte_04/1 -> Column_5(1B)/1
  Byte_01/1 -> Column_2(1B)/1
  Byte_07/1 -> Column_8(1B)/1
  Byte_03/1 -> Column_4(1B)/1
  Byte_06/1 -> Column_7(1B)/1
  Byte_1/1 -> Column_1(1B)/1
  Byte_02/1 -> Column_3(1B)/1

== system Computer_Library/Character_Table/Characters(Q..ARROW_UP)/Char_EQUAL ==
  Byte_01 : Constant  Value=char(2, EQUAL)  OutDataTypeStr=uint8
  Byte_02 : Constant  Value=char(3, EQUAL)  OutDataTypeStr=uint8
  Byte_03 : Constant  Value=char(4, EQUAL)  OutDataTypeStr=uint8
  Byte_04 : Constant  Value=char(5, EQUAL)  OutDataTypeStr=uint8
  Byte_05 : Constant  Value=char(6, EQUAL)  OutDataTypeStr=uint8
  Byte_06 : Constant  Value=char(7, EQUAL)  OutDataTypeStr=uint8
  Byte_07 : Constant  Value=char(8, EQUAL)  OutDataTypeStr=uint8
  Byte_1 : Constant  Value=char(1, EQUAL)  OutDataTypeStr=uint8
  Column_1(1B) : Outport
  Column_2(1B) : Outport  Port=2
  Column_3(1B) : Outport  Port=3
  Column_4(1B) : Outport  Port=4
  Column_5(1B) : Outport  Port=5
  Column_6(1B) : Outport  Port=6
  Column_7(1B) : Outport  Port=7
  Column_8(1B) : Outport  Port=8
  wires:
  Byte_05/1 -> Column_6(1B)/1
  Byte_04/1 -> Column_5(1B)/1
  Byte_01/1 -> Column_2(1B)/1
  Byte_07/1 -> Column_8(1B)/1
  Byte_03/1 -> Column_4(1B)/1
  Byte_06/1 -> Column_7(1B)/1
  Byte_1/1 -> Column_1(1B)/1
  Byte_02/1 -> Column_3(1B)/1

== system Computer_Library/Character_Table/Characters(Q..ARROW_UP)/Char_GREATER_THAN ==
  Byte_01 : Constant  Value=char(2, GREATER_THAN)  OutDataTypeStr=uint8
  Byte_02 : Constant  Value=char(3, GREATER_THAN)  OutDataTypeStr=uint8
  Byte_03 : Constant  Value=char(4, GREATER_THAN)  OutDataTypeStr=uint8
  Byte_04 : Constant  Value=char(5, GREATER_THAN)  OutDataTypeStr=uint8
  Byte_05 : Constant  Value=char(6, GREATER_THAN)  OutDataTypeStr=uint8
  Byte_06 : Constant  Value=char(7, GREATER_THAN)  OutDataTypeStr=uint8
  Byte_07 : Constant  Value=char(8, GREATER_THAN)  OutDataTypeStr=uint8
  Byte_1 : Constant  Value=char(1, GREATER_THAN)  OutDataTypeStr=uint8
  Column_1(1B) : Outport
  Column_2(1B) : Outport  Port=2
  Column_3(1B) : Outport  Port=3
  Column_4(1B) : Outport  Port=4
  Column_5(1B) : Outport  Port=5
  Column_6(1B) : Outport  Port=6
  Column_7(1B) : Outport  Port=7
  Column_8(1B) : Outport  Port=8
  wires:
  Byte_05/1 -> Column_6(1B)/1
  Byte_04/1 -> Column_5(1B)/1
  Byte_01/1 -> Column_2(1B)/1
  Byte_07/1 -> Column_8(1B)/1
  Byte_03/1 -> Column_4(1B)/1
  Byte_06/1 -> Column_7(1B)/1
  Byte_1/1 -> Column_1(1B)/1
  Byte_02/1 -> Column_3(1B)/1

== system Computer_Library/Character_Table/Characters(Q..ARROW_UP)/Char_LESS_THAN ==
  Byte_01 : Constant  Value=char(2, LESS_THAN)  OutDataTypeStr=uint8
  Byte_02 : Constant  Value=char(3, LESS_THAN)  OutDataTypeStr=uint8
  Byte_03 : Constant  Value=char(4, LESS_THAN)  OutDataTypeStr=uint8
  Byte_04 : Constant  Value=char(5, LESS_THAN)  OutDataTypeStr=uint8
  Byte_05 : Constant  Value=char(6, LESS_THAN)  OutDataTypeStr=uint8
  Byte_06 : Constant  Value=char(7, LESS_THAN)  OutDataTypeStr=uint8
  Byte_07 : Constant  Value=char(8, LESS_THAN)  OutDataTypeStr=uint8
  Byte_1 : Constant  Value=char(1, LESS_THAN)  OutDataTypeStr=uint8
  Column_1(1B) : Outport
  Column_2(1B) : Outport  Port=2
  Column_3(1B) : Outport  Port=3
  Column_4(1B) : Outport  Port=4
  Column_5(1B) : Outport  Port=5
  Column_6(1B) : Outport  Port=6
  Column_7(1B) : Outport  Port=7
  Column_8(1B) : Outport  Port=8
  wires:
  Byte_05/1 -> Column_6(1B)/1
  Byte_04/1 -> Column_5(1B)/1
  Byte_01/1 -> Column_2(1B)/1
  Byte_07/1 -> Column_8(1B)/1
  Byte_03/1 -> Column_4(1B)/1
  Byte_06/1 -> Column_7(1B)/1
  Byte_1/1 -> Column_1(1B)/1
  Byte_02/1 -> Column_3(1B)/1

== system Computer_Library/Character_Table/Characters(Q..ARROW_UP)/Char_MINUS ==
  Byte_01 : Constant  Value=char(2, MINUS)  OutDataTypeStr=uint8
  Byte_02 : Constant  Value=char(3, MINUS)  OutDataTypeStr=uint8
  Byte_03 : Constant  Value=char(4, MINUS)  OutDataTypeStr=uint8
  Byte_04 : Constant  Value=char(5, MINUS)  OutDataTypeStr=uint8
  Byte_05 : Constant  Value=char(6, MINUS)  OutDataTypeStr=uint8
  Byte_06 : Constant  Value=char(7, MINUS)  OutDataTypeStr=uint8
  Byte_07 : Constant  Value=char(8, MINUS)  OutDataTypeStr=uint8
  Byte_1 : Constant  Value=char(1, MINUS)  OutDataTypeStr=uint8
  Column_1(1B) : Outport
  Column_2(1B) : Outport  Port=2
  Column_3(1B) : Outport  Port=3
  Column_4(1B) : Outport  Port=4
  Column_5(1B) : Outport  Port=5
  Column_6(1B) : Outport  Port=6
  Column_7(1B) : Outport  Port=7
  Column_8(1B) : Outport  Port=8
  wires:
  Byte_05/1 -> Column_6(1B)/1
  Byte_04/1 -> Column_5(1B)/1
  Byte_01/1 -> Column_2(1B)/1
  Byte_07/1 -> Column_8(1B)/1
  Byte_03/1 -> Column_4(1B)/1
  Byte_06/1 -> Column_7(1B)/1
  Byte_1/1 -> Column_1(1B)/1
  Byte_02/1 -> Column_3(1B)/1

== system Computer_Library/Character_Table/Characters(Q..ARROW_UP)/Char_PLUS ==
  Byte_01 : Constant  Value=char(2, PLUS)  OutDataTypeStr=uint8
  Byte_02 : Constant  Value=char(3, PLUS)  OutDataTypeStr=uint8
  Byte_03 : Constant  Value=char(4, PLUS)  OutDataTypeStr=uint8
  Byte_04 : Constant  Value=char(5, PLUS)  OutDataTypeStr=uint8
  Byte_05 : Constant  Value=char(6, PLUS)  OutDataTypeStr=uint8
  Byte_06 : Constant  Value=char(7, PLUS)  OutDataTypeStr=uint8
  Byte_07 : Constant  Value=char(8, PLUS)  OutDataTypeStr=uint8
  Byte_1 : Constant  Value=char(1, PLUS)  OutDataTypeStr=uint8
  Column_1(1B) : Outport
  Column_2(1B) : Outport  Port=2
  Column_3(1B) : Outport  Port=3
  Column_4(1B) : Outport  Port=4
  Column_5(1B) : Outport  Port=5
  Column_6(1B) : Outport  Port=6
  Column_7(1B) : Outport  Port=7
  Column_8(1B) : Outport  Port=8
  wires:
  Byte_05/1 -> Column_6(1B)/1
  Byte_04/1 -> Column_5(1B)/1
  Byte_01/1 -> Column_2(1B)/1
  Byte_07/1 -> Column_8(1B)/1
  Byte_03/1 -> Column_4(1B)/1
  Byte_06/1 -> Column_7(1B)/1
  Byte_1/1 -> Column_1(1B)/1
  Byte_02/1 -> Column_3(1B)/1

== system Computer_Library/Character_Table/Characters(Q..ARROW_UP)/Char_Q ==
  Byte_01 : Constant  Value=char(2, Q)  OutDataTypeStr=uint8
  Byte_02 : Constant  Value=char(3, Q)  OutDataTypeStr=uint8
  Byte_03 : Constant  Value=char(4, Q)  OutDataTypeStr=uint8
  Byte_04 : Constant  Value=char(5, Q)  OutDataTypeStr=uint8
  Byte_05 : Constant  Value=char(6, Q)  OutDataTypeStr=uint8
  Byte_06 : Constant  Value=char(7, Q)  OutDataTypeStr=uint8
  Byte_07 : Constant  Value=char(8, Q)  OutDataTypeStr=uint8
  Byte_1 : Constant  Value=char(1, Q)  OutDataTypeStr=uint8
  Column_1(1B) : Outport
  Column_2(1B) : Outport  Port=2
  Column_3(1B) : Outport  Port=3
  Column_4(1B) : Outport  Port=4
  Column_5(1B) : Outport  Port=5
  Column_6(1B) : Outport  Port=6
  Column_7(1B) : Outport  Port=7
  Column_8(1B) : Outport  Port=8
  wires:
  Byte_05/1 -> Column_6(1B)/1
  Byte_04/1 -> Column_5(1B)/1
  Byte_01/1 -> Column_2(1B)/1
  Byte_07/1 -> Column_8(1B)/1
  Byte_03/1 -> Column_4(1B)/1
  Byte_06/1 -> Column_7(1B)/1
  Byte_1/1 -> Column_1(1B)/1
  Byte_02/1 -> Column_3(1B)/1

== system Computer_Library/Character_Table/Characters(Q..ARROW_UP)/Char_SEMICOLON ==
  Byte_01 : Constant  Value=char(2, SEMICOLON)  OutDataTypeStr=uint8
  Byte_02 : Constant  Value=char(3, SEMICOLON)  OutDataTypeStr=uint8
  Byte_03 : Constant  Value=char(4, SEMICOLON)  OutDataTypeStr=uint8
  Byte_04 : Constant  Value=char(5, SEMICOLON)  OutDataTypeStr=uint8
  Byte_05 : Constant  Value=char(6, SEMICOLON)  OutDataTypeStr=uint8
  Byte_06 : Constant  Value=char(7, SEMICOLON)  OutDataTypeStr=uint8
  Byte_07 : Constant  Value=char(8, SEMICOLON)  OutDataTypeStr=uint8
  Byte_1 : Constant  Value=char(1, SEMICOLON)  OutDataTypeStr=uint8
  Column_1(1B) : Outport
  Column_2(1B) : Outport  Port=2
  Column_3(1B) : Outport  Port=3
  Column_4(1B) : Outport  Port=4
  Column_5(1B) : Outport  Port=5
  Column_6(1B) : Outport  Port=6
  Column_7(1B) : Outport  Port=7
  Column_8(1B) : Outport  Port=8
  wires:
  Byte_05/1 -> Column_6(1B)/1
  Byte_04/1 -> Column_5(1B)/1
  Byte_01/1 -> Column_2(1B)/1
  Byte_07/1 -> Column_8(1B)/1
  Byte_03/1 -> Column_4(1B)/1
  Byte_06/1 -> Column_7(1B)/1
  Byte_1/1 -> Column_1(1B)/1
  Byte_02/1 -> Column_3(1B)/1

== system Computer_Library/Character_Table/Characters(Q..ARROW_UP)/Char_SLASH ==
  Byte_01 : Constant  Value=char(2, SLASH)  OutDataTypeStr=uint8
  Byte_02 : Constant  Value=char(3, SLASH)  OutDataTypeStr=uint8
  Byte_03 : Constant  Value=char(4, SLASH)  OutDataTypeStr=uint8
  Byte_04 : Constant  Value=char(5, SLASH)  OutDataTypeStr=uint8
  Byte_05 : Constant  Value=char(6, SLASH)  OutDataTypeStr=uint8
  Byte_06 : Constant  Value=char(7, SLASH)  OutDataTypeStr=uint8
  Byte_07 : Constant  Value=char(8, SLASH)  OutDataTypeStr=uint8
  Byte_1 : Constant  Value=char(1, SLASH)  OutDataTypeStr=uint8
  Column_1(1B) : Outport
  Column_2(1B) : Outport  Port=2
  Column_3(1B) : Outport  Port=3
  Column_4(1B) : Outport  Port=4
  Column_5(1B) : Outport  Port=5
  Column_6(1B) : Outport  Port=6
  Column_7(1B) : Outport  Port=7
  Column_8(1B) : Outport  Port=8
  wires:
  Byte_05/1 -> Column_6(1B)/1
  Byte_04/1 -> Column_5(1B)/1
  Byte_01/1 -> Column_2(1B)/1
  Byte_07/1 -> Column_8(1B)/1
  Byte_03/1 -> Column_4(1B)/1
  Byte_06/1 -> Column_7(1B)/1
  Byte_1/1 -> Column_1(1B)/1
  Byte_02/1 -> Column_3(1B)/1

== system Computer_Library/Character_Table/Characters(Q..ARROW_UP)/Char_X ==
  Byte_01 : Constant  Value=char(2, X)  OutDataTypeStr=uint8
  Byte_02 : Constant  Value=char(3, X)  OutDataTypeStr=uint8
  Byte_03 : Constant  Value=char(4, X)  OutDataTypeStr=uint8
  Byte_04 : Constant  Value=char(5, X)  OutDataTypeStr=uint8
  Byte_05 : Constant  Value=char(6, X)  OutDataTypeStr=uint8
  Byte_06 : Constant  Value=char(7, X)  OutDataTypeStr=uint8
  Byte_07 : Constant  Value=char(8, X)  OutDataTypeStr=uint8
  Byte_1 : Constant  Value=char(1, X)  OutDataTypeStr=uint8
  Column_1(1B) : Outport
  Column_2(1B) : Outport  Port=2
  Column_3(1B) : Outport  Port=3
  Column_4(1B) : Outport  Port=4
  Column_5(1B) : Outport  Port=5
  Column_6(1B) : Outport  Port=6
  Column_7(1B) : Outport  Port=7
  Column_8(1B) : Outport  Port=8
  wires:
  Byte_05/1 -> Column_6(1B)/1
  Byte_04/1 -> Column_5(1B)/1
  Byte_01/1 -> Column_2(1B)/1
  Byte_07/1 -> Column_8(1B)/1
  Byte_03/1 -> Column_4(1B)/1
  Byte_06/1 -> Column_7(1B)/1
  Byte_1/1 -> Column_1(1B)/1
  Byte_02/1 -> Column_3(1B)/1

== system Computer_Library/Character_Table/Characters(Q..ARROW_UP)/Char_Y ==
  Byte_01 : Constant  Value=char(2, Y)  OutDataTypeStr=uint8
  Byte_02 : Constant  Value=char(3, Y)  OutDataTypeStr=uint8
  Byte_03 : Constant  Value=char(4, Y)  OutDataTypeStr=uint8
  Byte_04 : Constant  Value=char(5, Y)  OutDataTypeStr=uint8
  Byte_05 : Constant  Value=char(6, Y)  OutDataTypeStr=uint8
  Byte_06 : Constant  Value=char(7, Y)  OutDataTypeStr=uint8
  Byte_07 : Constant  Value=char(8, Y)  OutDataTypeStr=uint8
  Byte_1 : Constant  Value=char(1, Y)  OutDataTypeStr=uint8
  Column_1(1B) : Outport
  Column_2(1B) : Outport  Port=2
  Column_3(1B) : Outport  Port=3
  Column_4(1B) : Outport  Port=4
  Column_5(1B) : Outport  Port=5
  Column_6(1B) : Outport  Port=6
  Column_7(1B) : Outport  Port=7
  Column_8(1B) : Outport  Port=8
  wires:
  Byte_05/1 -> Column_6(1B)/1
  Byte_04/1 -> Column_5(1B)/1
  Byte_01/1 -> Column_2(1B)/1
  Byte_07/1 -> Column_8(1B)/1
  Byte_03/1 -> Column_4(1B)/1
  Byte_06/1 -> Column_7(1B)/1
  Byte_1/1 -> Column_1(1B)/1
  Byte_02/1 -> Column_3(1B)/1

== system Computer_Library/Character_Table/Characters(Q..ARROW_UP)/Char_Z ==
  Byte_01 : Constant  Value=char(2, Z)  OutDataTypeStr=uint8
  Byte_02 : Constant  Value=char(3, Z)  OutDataTypeStr=uint8
  Byte_03 : Constant  Value=char(4, Z)  OutDataTypeStr=uint8
  Byte_04 : Constant  Value=char(5, Z)  OutDataTypeStr=uint8
  Byte_05 : Constant  Value=char(6, Z)  OutDataTypeStr=uint8
  Byte_06 : Constant  Value=char(7, Z)  OutDataTypeStr=uint8
  Byte_07 : Constant  Value=char(8, Z)  OutDataTypeStr=uint8
  Byte_1 : Constant  Value=char(1, Z)  OutDataTypeStr=uint8
  Column_1(1B) : Outport
  Column_2(1B) : Outport  Port=2
  Column_3(1B) : Outport  Port=3
  Column_4(1B) : Outport  Port=4
  Column_5(1B) : Outport  Port=5
  Column_6(1B) : Outport  Port=6
  Column_7(1B) : Outport  Port=7
  Column_8(1B) : Outport  Port=8
  wires:
  Byte_05/1 -> Column_6(1B)/1
  Byte_04/1 -> Column_5(1B)/1
  Byte_01/1 -> Column_2(1B)/1
  Byte_07/1 -> Column_8(1B)/1
  Byte_03/1 -> Column_4(1B)/1
  Byte_06/1 -> Column_7(1B)/1
  Byte_1/1 -> Column_1(1B)/1
  Byte_02/1 -> Column_3(1B)/1
